simulink model "IP_SwingUp_Design1"  (R2021a)
settings: Solver=VariableStepAuto  StartTime=0.0  StopTime=50  FixedStep=0.01  RelTol=1e-3
values from neighbouring files (symbols this model uses):
  b = 0.0    (= 0)    [Init_Setup_LQRArd.m]
  c = 1.91    [Init_Setup_LQRArd.m]
  Er = 2*m*g*l    (= 0.35789128452)    [Init_Setup_LQRArd.m]
  g = 9.81    [Init_Setup_LQRArd.m]
  I = 0.00527    [Init_Setup_LQRArd.m]
  kcw = 1.5    [Init_Setup_LQRArd.m]
  kem = 1.5    [Init_Setup_LQRArd.m]
  KK = lqr(A,B,Q,R)    [Init_Setup_LQRArd.m]
  ksu = 1.5    [Init_Setup_LQRArd.m]
  kvw = 0.75    [Init_Setup_LQRArd.m]
  l = 0.26322    [Init_Setup_LQRArd.m]
  Lmax = 0.2    [Init_Setup_LQRArd.m]
  M = 0.25    [Init_Setup_LQRArd.m]
  m = 0.0693    [Init_Setup_LQRArd.m]
  M_c = 0.25    [Init_Setup_LQRArd.m]
  n = 1.05    [Init_Setup_LQRArd.m]
  Vmax = 0.5    [Init_Setup_LQRArd.m]
settings Model: Creator=jitendra  LastModifiedBy=M7540
settings SolverCC: AlgebraicLoopSolver=LineSearch
settings DataIOCC: ExternalInput=getinputstruct(op_trim1)  InitialState=getstatestruct(op_trim1)  ReturnWorkspaceOutputs=off
settings DebuggingCC: SFMachineParentedDataDiag=warning  ArithmeticOperatorsInVariantConditions=warning
settings SFSimCC: SimUseLocalCustomCode=off  CustomCodeUndefinedFunction=UseInterfaceOnly
settings RTWCC: RTWUseLocalCustomCode=off

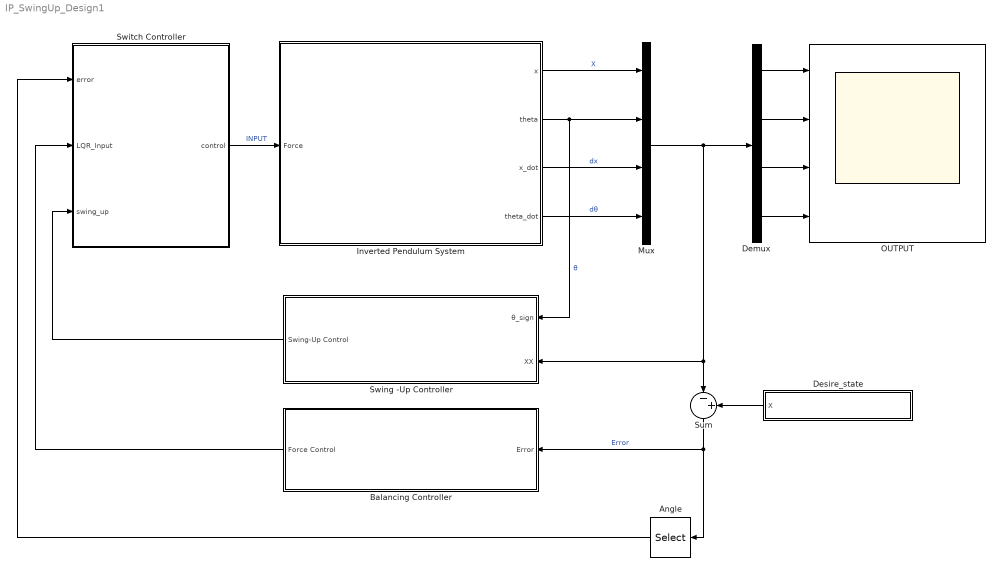
== system IP_SwingUp_Design1 ==
  Angle : Selector  InputPortWidth=4  IndexOptions=Index vector (dialog)  Indices=[2]  OutputSizes=1
  Balancing Controller : Subsystem
  Demux : Demux
  Desire_state : Subsystem
  Inverted Pendulum System : Subsystem
      mask Display: image('C:\Users\M7540\Desktop\ip\Image\mô hình toán học con lắc.jpg'); % Use "Edit Image" on toolstrip to change.
  Mux : Mux
  OUTPUT : Scope  NumInputPorts=4
  Sum : Sum  Inputs=|-+
  Swing -Up Controller : Subsystem
  Switch Controller : Subsystem
  wires:
  Inverted Pendulum System/3(x_dot) -> Mux/3  "dx"
  Inverted Pendulum System/1(x) -> Mux/1  "X"
  Inverted Pendulum System/4(theta_dot) -> Mux/4  "dθ"
  Mux/1 -> Demux/1, Sum/1, Swing -Up Controller/2(XX)
  Desire_state/1(X) -> Sum/2
  Demux/1 -> OUTPUT/1
  Demux/3 -> OUTPUT/3
  Demux/2 -> OUTPUT/2
  Inverted Pendulum System/2(theta) -> Swing -Up Controller/1(θ_sign), Mux/2  "θ"
  Demux/4 -> OUTPUT/4
  Switch Controller/1(control) -> Inverted Pendulum System/1(Force)  "INPUT"
  Sum/1 -> Angle/1, Balancing Controller/1(Error)  "Error"
  Balancing Controller/1(Force Control) -> Switch Controller/2("LQR_Input ")
  Swing -Up Controller/1(Swing-Up Control) -> Switch Controller/3(swing_up)
  Angle/1 -> Switch Controller/1(error)

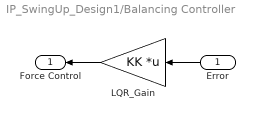
== system IP_SwingUp_Design1/Balancing Controller ==
  Error : Inport
  LQR_Gain : Gain  Gain=KK  Multiplication=Matrix(K*u)
  Force Control : Outport
  wires:
  LQR_Gain/1 -> Force Control/1
  Error/1 -> LQR_Gain/1

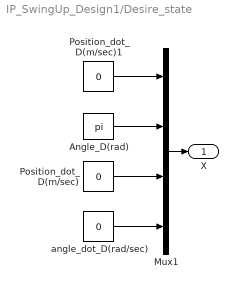
== system IP_SwingUp_Design1/Desire_state ==
  Angle_D(rad) : Constant  Value=pi
  Mux1 : Mux
  Position_dot_D(m/sec) : Constant  Value=0
  Position_dot_D(m/sec)1 : Constant  Value=0
  angle_dot_D(rad/sec) : Constant  Value=0
  X : Outport  VectorParamsAs1DForOutWhenUnconnected=off
  wires:
  Mux1/1 -> X/1
  Position_dot_D(m/sec)/1 -> Mux1/3
  angle_dot_D(rad/sec)/1 -> Mux1/4
  Angle_D(rad)/1 -> Mux1/2
  Position_dot_D(m/sec)1/1 -> Mux1/1

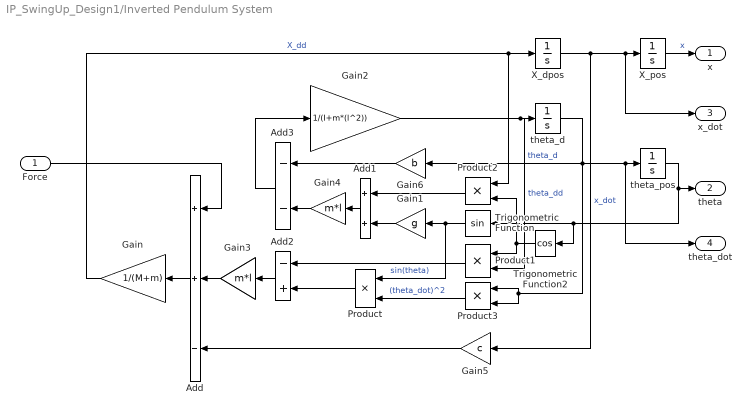
== system IP_SwingUp_Design1/Inverted Pendulum System ==
  Force : Inport
  Add : Sum  Inputs=++-
  Add1 : Sum
  Add2 : Sum  Inputs=-+
  Add3 : Sum  Inputs=--
  Gain : Gain  Gain=1/(M+m)
  Gain1 : Gain  Gain=g
  Gain2 : Gain  Gain=1/(I+m*(l^2))
  Gain3 : Gain  Gain=m*l
  Gain4 : Gain  Gain=m*l
  Gain5 : Gain  Gain=c
  Gain6 : Gain  Gain=b
  Product{,1..3} (4 alike) : Product
  Trigonometric Function : Trigonometry
  Trigonometric Function2 : Trigonometry  Operator=cos
  X_dpos : Integrator  InitialCondition=0.01
  X_pos : Integrator  InitialCondition=0.0
  theta_d : Integrator
  theta_pos : Integrator  InitialCondition=-0.001*(pi/180)
  x : Outport  VectorParamsAs1DForOutWhenUnconnected=off
  theta : Outport  Port=2  VectorParamsAs1DForOutWhenUnconnected=off
  x_dot : Outport  Port=3  VectorParamsAs1DForOutWhenUnconnected=off
  theta_dot : Outport  Port=4  VectorParamsAs1DForOutWhenUnconnected=off
  wires:
  Gain5/1 -> Add/3
  Add2/1 -> Gain3/1
  Add3/1 -> Gain2/1
  Trigonometric Function2/1 -> Product2/2, Product1/1
  Trigonometric Function/1 -> Product/1, Gain1/1  "sin(theta)"
  Gain3/1 -> Add/2
  theta_d/1 -> Product3/2, Product3/1, Gain6/1, theta_dot/1, theta_pos/1  "theta_d"
  Product2/1 -> Add1/1
  Product/1 -> Add2/2
  Gain4/1 -> Add3/2
  Product3/1 -> Product/2  "(theta_dot)^2"
  X_pos/1 -> x/1  "x"
  Product1/1 -> Add2/1
  Gain/1 -> X_dpos/1, Product2/1  "X_dd"
  Add/1 -> Gain/1
  Gain2/1 -> Product1/2, theta_d/1  "theta_dd"
  Gain6/1 -> Add3/1
  theta_pos/1 -> Trigonometric Function2/1, Trigonometric Function/1, theta/1
  Force/1 -> Add/1
  Gain1/1 -> Add1/2
  X_dpos/1 -> x_dot/1, X_pos/1, Gain5/1  "x_dot"
  Add1/1 -> Gain4/1

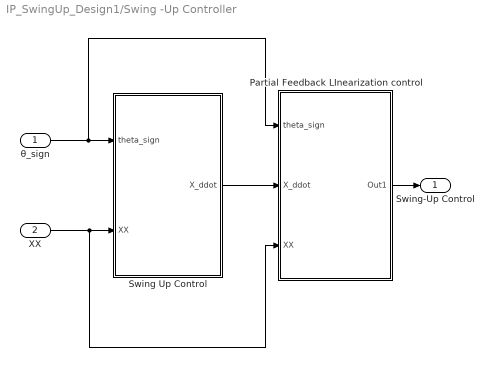
== system IP_SwingUp_Design1/Swing -Up Controller ==
  θ_sign : Inport
  XX : Inport  Port=2
  Partial Feedback LInearization control : Subsystem
  Swing Up Control : Subsystem
  Swing-Up Control : Outport
  wires:
  XX/1 -> Swing Up Control/2(XX), Partial Feedback LInearization control/3(XX)
  Partial Feedback LInearization control/1(Out1) -> Swing-Up Control/1
  θ_sign/1 -> Swing Up Control/1(theta_sign), Partial Feedback LInearization control/1(theta_sign)
  Swing Up Control/1(X_ddot) -> Partial Feedback LInearization control/2(X_ddot)

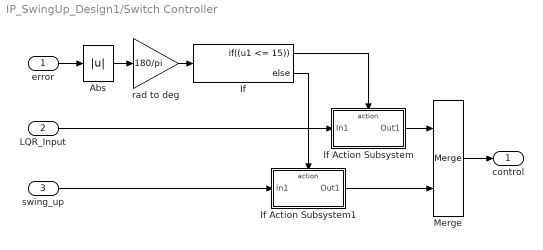
== system IP_SwingUp_Design1/Switch Controller ==
  error : Inport
  "LQR_Input " : Inport  Port=2
  swing_up : Inport  Port=3
  Abs : Abs
  If : If  IfExpression=(u1 <= 15)
  If Action Subsystem : Subsystem  TreatAsAtomicUnit=on
  If Action Subsystem1 : Subsystem  TreatAsAtomicUnit=on
  Merge : Merge
  rad to deg : Gain  Gain=180/pi
  control : Outport  VectorParamsAs1DForOutWhenUnconnected=off
  wires:
  Merge/1 -> control/1
  If/1 -> If Action Subsystem/Action
  If/2 -> If Action Subsystem1/Action
  swing_up/1 -> If Action Subsystem1/1(In1)
  If Action Subsystem1/1(Out1) -> Merge/2
  error/1 -> Abs/1
  Abs/1 -> rad to deg/1
  rad to deg/1 -> If/1
  If Action Subsystem/1(Out1) -> Merge/1
  "LQR_Input "/1 -> If Action Subsystem/1(In1)

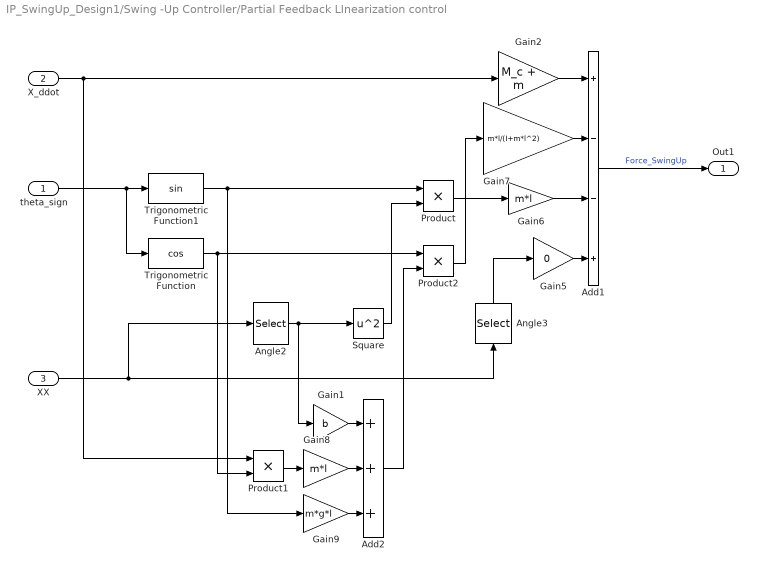
== system IP_SwingUp_Design1/Swing -Up Controller/Partial Feedback LInearization control ==
  theta_sign : Inport
  X_ddot : Inport  Port=2
  XX : Inport  Port=3
  Add1 : Sum  Inputs=+--+
  Add2 : Sum  Inputs=+++
  Angle2 : Selector  InputPortWidth=4  IndexOptions=Index vector (dialog)  Indices=[4]  OutputSizes=1
  Angle3 : Selector  InputPortWidth=4  IndexOptions=Index vector (dialog)  Indices=[3]  OutputSizes=1
  Gain1 : Gain  Gain=b
  Gain2 : Gain  Gain=M_c + m
  Gain5 : Gain  Gain=0
  Gain6 : Gain  Gain=m*l
  Gain7 : Gain  Gain=m*l/(I+m*l^2)
  Gain8 : Gain  Gain=m*l
  Gain9 : Gain  Gain=m*g*l
  Product : Product
  Product1 : Product
  Product2 : Product
  Square : Math  Operator=square  SignedPower=on  RndMeth=Zero  SaturateOnIntegerOverflow=on
  Trigonometric Function : Trigonometry  Operator=cos
  Trigonometric Function1 : Trigonometry
  Out1 : Outport  VectorParamsAs1DForOutWhenUnconnected=off
  wires:
  Angle3/1 -> Gain5/1
  X_ddot/1 -> Gain2/1, Product1/1
  Gain2/1 -> Add1/1
  Add1/1 -> Out1/1  "Force_SwingUp"
  Gain5/1 -> Add1/4
  Gain7/1 -> Add1/2
  theta_sign/1 -> Trigonometric Function/1, Trigonometric Function1/1
  XX/1 -> Angle3/1, Angle2/1
  Angle2/1 -> Square/1, Gain1/1
  Product/1 -> Gain6/1
  Trigonometric Function1/1 -> Product/1, Gain9/1
  Square/1 -> Product/2
  Gain6/1 -> Add1/3
  Gain1/1 -> Add2/1
  Product1/1 -> Gain8/1
  Trigonometric Function/1 -> Product2/1, Product1/2
  Gain8/1 -> Add2/2
  Gain9/1 -> Add2/3
  Add2/1 -> Product2/2
  Product2/1 -> Gain7/1

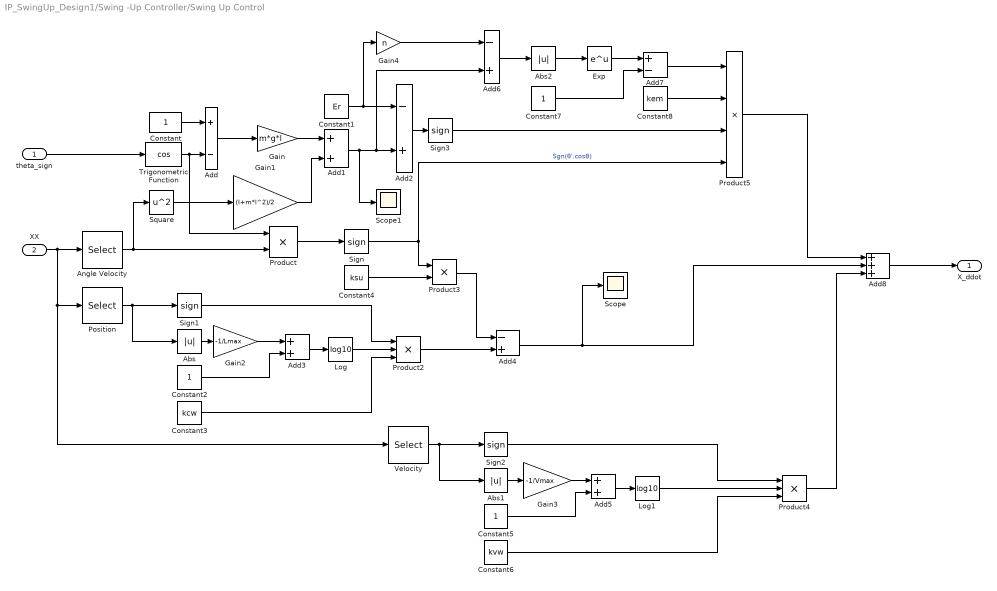
== system IP_SwingUp_Design1/Swing -Up Controller/Swing Up Control ==
  theta_sign : Inport
  XX : Inport  Port=2
  Abs : Abs
  Abs1 : Abs
  Abs2 : Abs
  Add : Sum  Inputs=+-
  Add1 : Sum
  Add2 : Sum  Inputs=-+
  Add3 : Sum
  Add4 : Sum  Inputs=-+
  Add5 : Sum
  Add6 : Sum  Inputs=-+
  Add7 : Sum  Inputs=+-
  Add8 : Sum  Inputs=3
  Angle Velocity : Selector  InputPortWidth=4  IndexOptions=Index vector (dialog)  Indices=[4]  OutputSizes=1
  Constant{,2,5,7} (4 alike) : Constant
  Constant1 : Constant  Value=Er
  Constant3 : Constant  Value=kcw
  Constant4 : Constant  Value=ksu
  Constant6 : Constant  Value=kvw
  Constant8 : Constant  Value=kem
  Exp : Math  SaturateOnIntegerOverflow=on
  Gain : Gain  Gain=m*g*l
  Gain1 : Gain  Gain=(I+m*l^2)/2
  Gain2 : Gain  Gain=-1/Lmax
  Gain3 : Gain  Gain=-1/Vmax
  Gain4 : Gain  Gain=n
  Log : Math  Operator=log10  SaturateOnIntegerOverflow=on
  Log1 : Math  Operator=log10  SaturateOnIntegerOverflow=on
  Position : Selector  InputPortWidth=4  IndexOptions=Index vector (dialog)  Indices=[1]  OutputSizes=1
  Product : Product
  Product2 : Product  Inputs=3
  Product3 : Product
  Product4 : Product  Inputs=3
  Product5 : Product  Inputs=4
  Scope : Scope
  Scope1 : Scope
  Sign{,1..3} (4 alike) : Signum
  Square : Math  Operator=square  SignedPower=on  RndMeth=Zero  SaturateOnIntegerOverflow=on
  Trigonometric Function : Trigonometry  Operator=cos
  Velocity : Selector  InputPortWidth=4  IndexOptions=Index vector (dialog)  Indices=[3]  OutputSizes=1
  X_ddot : Outport
  wires:
  Constant/1 -> Add/1
  Add/1 -> Gain/1
  Trigonometric Function/1 -> Product/1, Add/2
  Square/1 -> Gain1/1
  XX/1 -> Velocity/1, Position/1, Angle Velocity/1
  Gain/1 -> Add1/1
  Gain1/1 -> Add1/2
  Product/1 -> Sign/1
  Add1/1 -> Scope1/1, Add6/2, Add2/2
  Sign/1 -> Product5/4, Product3/1  "Sgn(θ'.cosθ)"
  theta_sign/1 -> Trigonometric Function/1
  Constant1/1 -> Gain4/1, Add2/1
  Angle Velocity/1 -> Product/2, Square/1
  Position/1 -> Abs/1, Sign1/1
  Abs/1 -> Gain2/1
  Gain2/1 -> Add3/1
  Constant2/1 -> Add3/2
  Add3/1 -> Log/1
  Sign1/1 -> Product2/1
  Log/1 -> Product2/2
  Constant3/1 -> Product2/3
  Constant4/1 -> Product3/2
  Product3/1 -> Add4/1
  Product2/1 -> Add4/2
  Abs1/1 -> Gain3/1
  Gain3/1 -> Add5/1
  Add5/1 -> Log1/1
  Constant5/1 -> Add5/2
  Velocity/1 -> Abs1/1, Sign2/1
  Sign2/1 -> Product4/1
  Log1/1 -> Product4/2
  Constant6/1 -> Product4/3
  Add2/1 -> Sign3/1
  Gain4/1 -> Add6/1
  Add6/1 -> Abs2/1
  Abs2/1 -> Exp/1
  Exp/1 -> Add7/1
  Constant7/1 -> Add7/2
  Add7/1 -> Product5/1
  Constant8/1 -> Product5/2
  Sign3/1 -> Product5/3
  Product5/1 -> Add8/1
  Add4/1 -> Scope/1, Add8/2
  Product4/1 -> Add8/3
  Add8/1 -> X_ddot/1

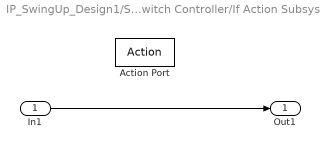
== system IP_SwingUp_Design1/Switch Controller/If Action Subsystem ==
  In1 : Inport
  Action Port : ActionPort  ActionPortLabel=if((u1 <= 15))
  Out1 : Outport  VectorParamsAs1DForOutWhenUnconnected=off
  wires:
  In1/1 -> Out1/1

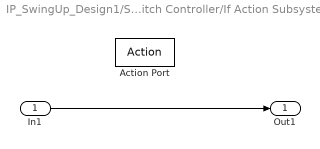
== system IP_SwingUp_Design1/Switch Controller/If Action Subsystem1 ==
  In1 : Inport
  Action Port : ActionPort  ActionPortLabel=else
  Out1 : Outport  VectorParamsAs1DForOutWhenUnconnected=off
  wires:
  In1/1 -> Out1/1
